simulink model "Lab3_Sim"  (R2024a)
settings: Solver=VariableStepAuto  StartTime=0.0  StopTime=60480000  RelTol=1e-3
values from neighbouring files (symbols this model uses):
  G = 6.674e-11    [L_points.m]    (also in Lab3_Driver.m; Lab5.m; Lab8.m; LagrangePoints.m = 6.67408e-11)
  Mm = 6.4171e23    (= 6.4171e+23)    [Lab3_Driver.m]    (also in LagrangePoints.m = 7.34767309e+22)
  Mp = 5.97219e24    (= 5.97219e+24)    [Lab3_Driver.m]
  Ms = 1988410e24    (= 1.98841e+30)    [Lab3_Driver.m]    (also in LagrangePoints.m = 5.97219e+24)
  Pos_m = [-2.299762717931310E+08 9.863481268283156E+07 7.712126942588501E+06]*1000    [Lab3_Driver.m]
  Pos_p = [-5.328792362541436E+07 -1.426707827423932E+08 3.981048565176874E+04]*1000    [Lab3_Driver.m]
  Pos_s = [-1.313e6 -1.803e5 -4.319e4]*1000    [Lab3_Driver.m]
  Pos_v = [-5.362193933254258E+07 -1.428620826284412E+08 4.195466200186312E+04]*1000    [Lab3_Driver.m]
  Vel_m = [-8.699321075487822E+00 -2.018860873085168E+01 -2.092884078165804E-01]*1000    [Lab3_Driver.m]
  Vel_p = [2.749848392692773E+01 -1.032646088959717E+01 1.535581598741675E-03]*1000    [Lab3_Driver.m]
  Vel_s = [4.508e-3 -1.335e-2 -5.769e-3]*1000    [Lab3_Driver.m]
  Vel_v = [-2.625497707637767E+01 1.649830245531765E+01 5.627457721235540E-02]*1000    [Lab3_Driver.m]
settings Model: Creator=sgtjake2  LastModifiedBy=Thomas
settings SolverCC: InitialStep=3600

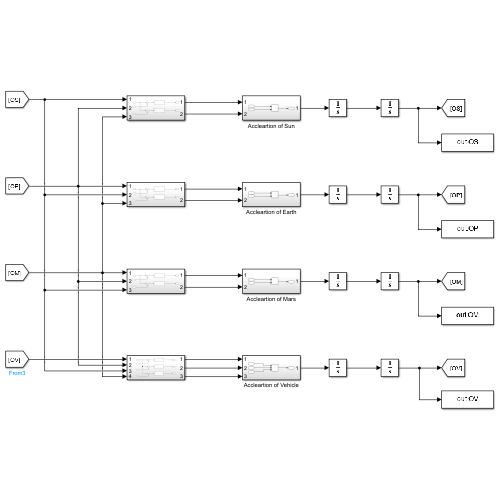
[thumbnail: Simulink's stored preview of the top-level diagram]
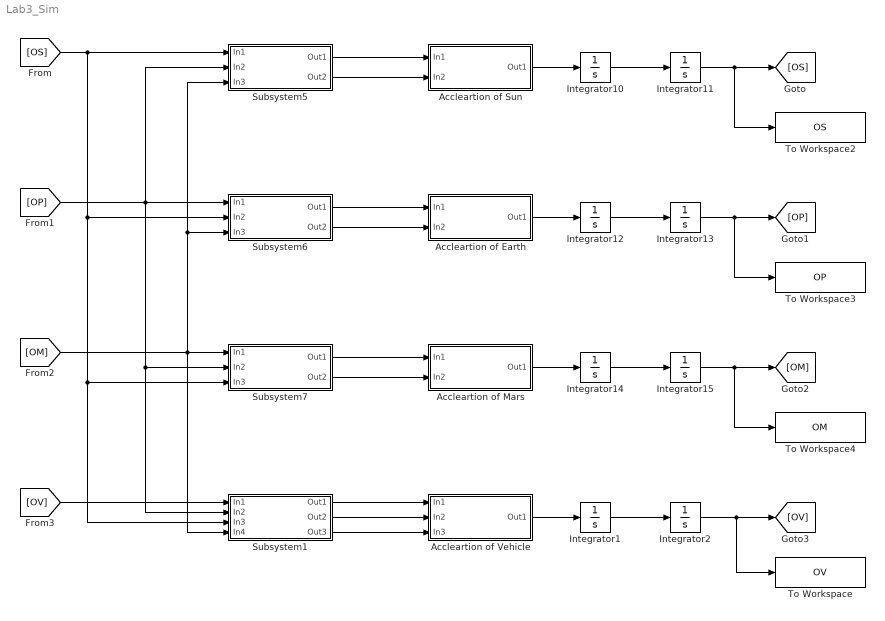
== system Lab3_Sim ==
  Accleartion of Earth : Subsystem
  Accleartion of Mars : Subsystem
  Accleartion of Sun : Subsystem
  Accleartion of Vehicle : Subsystem
  Integrator1 : Integrator  InitialCondition=Vel_v
  Integrator10 : Integrator  InitialCondition=Vel_s
  Integrator11 : Integrator  InitialCondition=Pos_s
  Integrator12 : Integrator  InitialCondition=Vel_p
  Integrator13 : Integrator  InitialCondition=Pos_p
  Integrator14 : Integrator  InitialCondition=Vel_m
  Integrator15 : Integrator  InitialCondition=Pos_m
  Integrator2 : Integrator  InitialCondition=Pos_v
  Subsystem1 : Subsystem
  Subsystem5 : Subsystem
  Subsystem6 : Subsystem
  Subsystem7 : Subsystem
  To Workspace : ToWorkspace  VariableName=OV  SaveFormat=Timeseries  SampleTime=-1
  To Workspace2 : ToWorkspace  VariableName=OS  SaveFormat=Timeseries  SampleTime=-1
  To Workspace3 : ToWorkspace  VariableName=OP  SaveFormat=Timeseries  SampleTime=3600
  To Workspace4 : ToWorkspace  VariableName=OM  SaveFormat=Timeseries  SampleTime=-1
  wires:
  Accleartion of Sun/1(Out1) -> Integrator10/1
  Integrator10/1 -> Integrator11/1
  Subsystem5/1(Out1) -> Accleartion of Sun/1(In1)
  Subsystem5/2(Out2) -> Accleartion of Sun/2(In2)
  Integrator11/1 -> To Workspace2/1, [OS]
  [OS] -> Subsystem1/3(In3), Subsystem7/3(In3), Subsystem6/2(In2), Subsystem5/1(In1)
  Accleartion of Earth/1(Out1) -> Integrator12/1
  Subsystem6/2(Out2) -> Accleartion of Earth/2(In2)
  Integrator12/1 -> Integrator13/1
  Subsystem6/1(Out1) -> Accleartion of Earth/1(In1)
  Integrator13/1 -> To Workspace3/1, [OP]
  [OP] -> Subsystem1/2(In2), Subsystem7/2(In2), Subsystem5/2(In2), Subsystem6/1(In1)
  Accleartion of Mars/1(Out1) -> Integrator14/1
  Subsystem7/2(Out2) -> Accleartion of Mars/2(In2)
  Integrator14/1 -> Integrator15/1
  Subsystem7/1(Out1) -> Accleartion of Mars/1(In1)
  Integrator15/1 -> To Workspace4/1, [OM]
  [OM] -> Subsystem5/3(In3), Subsystem6/3(In3), Subsystem1/4(In4), Subsystem7/1(In1)
  Integrator1/1 -> Integrator2/1
  Accleartion of Vehicle/1(Out1) -> Integrator1/1
  Integrator2/1 -> To Workspace/1, [OV]
  Subsystem1/1(Out1) -> Accleartion of Vehicle/1(In1)
  Subsystem1/2(Out2) -> Accleartion of Vehicle/2(In2)
  Subsystem1/3(Out3) -> Accleartion of Vehicle/3(In3)
  [OV] -> Subsystem1/1(In1)

== system Lab3_Sim/Accleartion of Earth ==
  In1 : Inport
  In2 : Inport  Port=2
  Add : Sum
  Out1 : Outport
  wires:
  Add/1 -> Out1/1
  In1/1 -> Add/1
  In2/1 -> Add/2

== system Lab3_Sim/Accleartion of Mars ==
  In1 : Inport
  In2 : Inport  Port=2
  Add : Sum
  Out1 : Outport
  wires:
  Add/1 -> Out1/1
  In1/1 -> Add/1
  In2/1 -> Add/2

== system Lab3_Sim/Accleartion of Sun ==
  In1 : Inport
  In2 : Inport  Port=2
  Add : Sum
  Out1 : Outport
  wires:
  Add/1 -> Out1/1
  In1/1 -> Add/1
  In2/1 -> Add/2

== system Lab3_Sim/Accleartion of Vehicle ==
  In1 : Inport
  In2 : Inport  Port=2
  In3 : Inport  Port=3
  Add : Sum  Inputs=+++
  Out1 : Outport
  wires:
  Add/1 -> Out1/1
  In1/1 -> Add/1
  In2/1 -> Add/2
  In3/1 -> Add/3

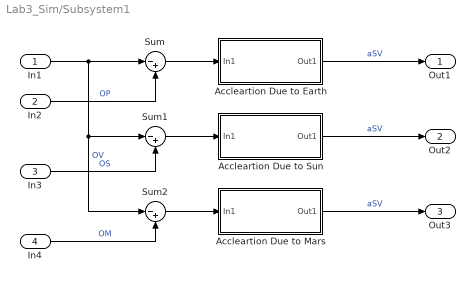
== system Lab3_Sim/Subsystem1 ==
  In1 : Inport
  In2 : Inport  Port=2
  In3 : Inport  Port=3
  In4 : Inport  Port=4
  Accleartion Due to Earth : Subsystem
  Accleartion Due to Mars : Subsystem
  Accleartion Due to Sun : Subsystem
  Sum : Sum  Inputs=|-+
  Sum1 : Sum  Inputs=|-+
  Sum2 : Sum  Inputs=|-+
  Out1 : Outport
  Out2 : Outport  Port=2
  Out3 : Outport  Port=3
  wires:
  Accleartion Due to Earth/1(Out1) -> Out1/1  "aSV"
  Accleartion Due to Sun/1(Out1) -> Out2/1  "aSV"
  Sum/1 -> Accleartion Due to Earth/1(In1)
  Sum1/1 -> Accleartion Due to Sun/1(In1)
  In1/1 -> Sum2/1, Sum1/1, Sum/1  "OV"
  In2/1 -> Sum/2  "OP"
  In3/1 -> Sum1/2  "OS"
  Accleartion Due to Mars/1(Out1) -> Out3/1  "aSV"
  Sum2/1 -> Accleartion Due to Mars/1(In1)
  In4/1 -> Sum2/2  "OM"

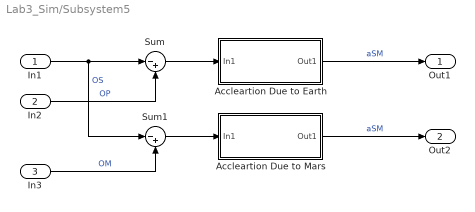
== system Lab3_Sim/Subsystem5 ==
  In1 : Inport
  In2 : Inport  Port=2
  In3 : Inport  Port=3
  Accleartion Due to Earth : Subsystem
  Accleartion Due to Mars : Subsystem
  Sum : Sum  Inputs=|-+
  Sum1 : Sum  Inputs=|-+
  Out1 : Outport
  Out2 : Outport  Port=2
  wires:
  Accleartion Due to Earth/1(Out1) -> Out1/1  "aSM"
  Accleartion Due to Mars/1(Out1) -> Out2/1  "aSM"
  Sum/1 -> Accleartion Due to Earth/1(In1)
  Sum1/1 -> Accleartion Due to Mars/1(In1)
  In1/1 -> Sum1/1, Sum/1  "OS"
  In2/1 -> Sum/2  "OP"
  In3/1 -> Sum1/2  "OM"

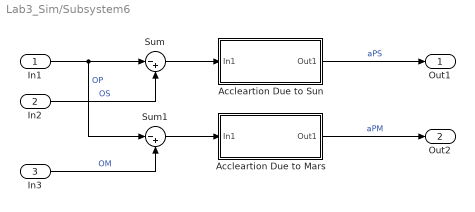
== system Lab3_Sim/Subsystem6 ==
  In1 : Inport
  In2 : Inport  Port=2
  In3 : Inport  Port=3
  Accleartion Due to Mars : Subsystem
  Accleartion Due to Sun : Subsystem
  Sum : Sum  Inputs=|-+
  Sum1 : Sum  Inputs=|-+
  Out1 : Outport
  Out2 : Outport  Port=2
  wires:
  Accleartion Due to Sun/1(Out1) -> Out1/1  "aPS"
  Accleartion Due to Mars/1(Out1) -> Out2/1  "aPM"
  Sum/1 -> Accleartion Due to Sun/1(In1)
  Sum1/1 -> Accleartion Due to Mars/1(In1)
  In1/1 -> Sum1/1, Sum/1  "OP"
  In2/1 -> Sum/2  "OS"
  In3/1 -> Sum1/2  "OM"

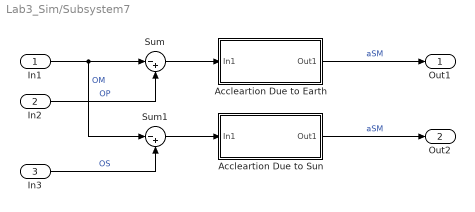
== system Lab3_Sim/Subsystem7 ==
  In1 : Inport
  In2 : Inport  Port=2
  In3 : Inport  Port=3
  Accleartion Due to Earth : Subsystem
  Accleartion Due to Sun : Subsystem
  Sum : Sum  Inputs=|-+
  Sum1 : Sum  Inputs=|-+
  Out1 : Outport
  Out2 : Outport  Port=2
  wires:
  Accleartion Due to Earth/1(Out1) -> Out1/1  "aSM"
  Accleartion Due to Sun/1(Out1) -> Out2/1  "aSM"
  Sum/1 -> Accleartion Due to Earth/1(In1)
  Sum1/1 -> Accleartion Due to Sun/1(In1)
  In1/1 -> Sum1/1, Sum/1  "OM"
  In2/1 -> Sum/2  "OP"
  In3/1 -> Sum1/2  "OS"

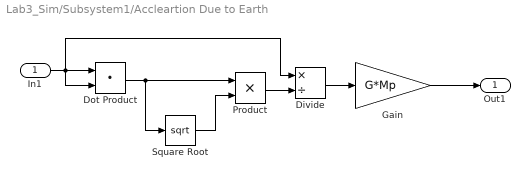
== system Lab3_Sim/Subsystem1/Accleartion Due to Earth ==
  In1 : Inport
  Divide : Product  Inputs=*/
  Dot Product : DotProduct  OutDataTypeStr=Inherit: Inherit via internal rule
  Gain : Gain  Gain=G*Mp
  Product : Product
  Square Root : Sqrt
  Out1 : Outport
  wires:
  In1/1 -> Divide/1, Dot Product/2, Dot Product/1
  Dot Product/1 -> Square Root/1, Product/1
  Square Root/1 -> Product/2
  Product/1 -> Divide/2
  Gain/1 -> Out1/1
  Divide/1 -> Gain/1

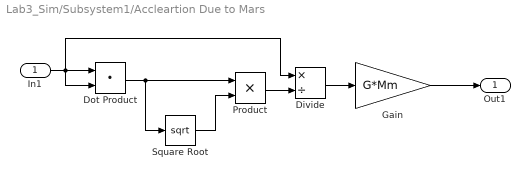
== system Lab3_Sim/Subsystem1/Accleartion Due to Mars ==
  In1 : Inport
  Divide : Product  Inputs=*/
  Dot Product : DotProduct  OutDataTypeStr=Inherit: Inherit via internal rule
  Gain : Gain  Gain=G*Mm
  Product : Product
  Square Root : Sqrt
  Out1 : Outport
  wires:
  In1/1 -> Divide/1, Dot Product/2, Dot Product/1
  Dot Product/1 -> Square Root/1, Product/1
  Square Root/1 -> Product/2
  Product/1 -> Divide/2
  Gain/1 -> Out1/1
  Divide/1 -> Gain/1

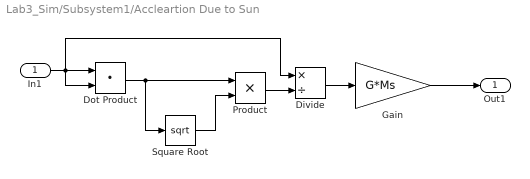
== system Lab3_Sim/Subsystem1/Accleartion Due to Sun ==
  In1 : Inport
  Divide : Product  Inputs=*/
  Dot Product : DotProduct  OutDataTypeStr=Inherit: Inherit via internal rule
  Gain : Gain  Gain=G*Ms
  Product : Product
  Square Root : Sqrt
  Out1 : Outport
  wires:
  In1/1 -> Divide/1, Dot Product/2, Dot Product/1
  Dot Product/1 -> Square Root/1, Product/1
  Square Root/1 -> Product/2
  Product/1 -> Divide/2
  Gain/1 -> Out1/1
  Divide/1 -> Gain/1

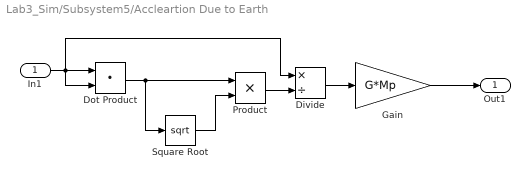
== system Lab3_Sim/Subsystem5/Accleartion Due to Earth ==
  In1 : Inport
  Divide : Product  Inputs=*/
  Dot Product : DotProduct  OutDataTypeStr=Inherit: Inherit via internal rule
  Gain : Gain  Gain=G*Mp
  Product : Product
  Square Root : Sqrt
  Out1 : Outport
  wires:
  In1/1 -> Divide/1, Dot Product/2, Dot Product/1
  Dot Product/1 -> Square Root/1, Product/1
  Square Root/1 -> Product/2
  Product/1 -> Divide/2
  Gain/1 -> Out1/1
  Divide/1 -> Gain/1

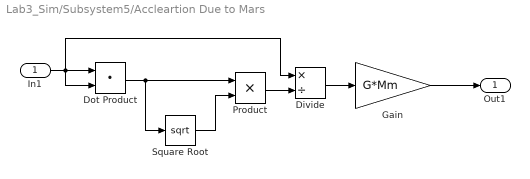
== system Lab3_Sim/Subsystem5/Accleartion Due to Mars ==
  In1 : Inport
  Divide : Product  Inputs=*/
  Dot Product : DotProduct  OutDataTypeStr=Inherit: Inherit via internal rule
  Gain : Gain  Gain=G*Mm
  Product : Product
  Square Root : Sqrt
  Out1 : Outport
  wires:
  In1/1 -> Divide/1, Dot Product/2, Dot Product/1
  Dot Product/1 -> Square Root/1, Product/1
  Square Root/1 -> Product/2
  Product/1 -> Divide/2
  Gain/1 -> Out1/1
  Divide/1 -> Gain/1

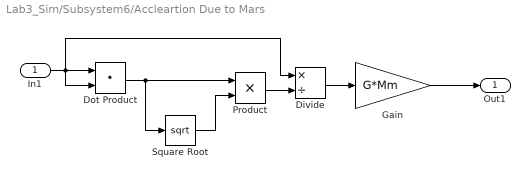
== system Lab3_Sim/Subsystem6/Accleartion Due to Mars ==
  In1 : Inport
  Divide : Product  Inputs=*/
  Dot Product : DotProduct  OutDataTypeStr=Inherit: Inherit via internal rule
  Gain : Gain  Gain=G*Mm
  Product : Product
  Square Root : Sqrt
  Out1 : Outport
  wires:
  In1/1 -> Divide/1, Dot Product/2, Dot Product/1
  Dot Product/1 -> Square Root/1, Product/1
  Square Root/1 -> Product/2
  Product/1 -> Divide/2
  Gain/1 -> Out1/1
  Divide/1 -> Gain/1

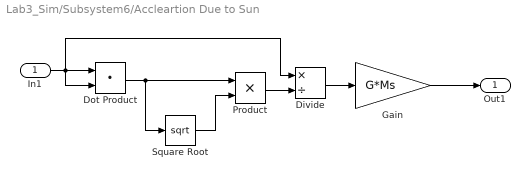
== system Lab3_Sim/Subsystem6/Accleartion Due to Sun ==
  In1 : Inport
  Divide : Product  Inputs=*/
  Dot Product : DotProduct  OutDataTypeStr=Inherit: Inherit via internal rule
  Gain : Gain  Gain=G*Ms
  Product : Product
  Square Root : Sqrt
  Out1 : Outport
  wires:
  In1/1 -> Divide/1, Dot Product/2, Dot Product/1
  Dot Product/1 -> Square Root/1, Product/1
  Square Root/1 -> Product/2
  Product/1 -> Divide/2
  Gain/1 -> Out1/1
  Divide/1 -> Gain/1

== system Lab3_Sim/Subsystem7/Accleartion Due to Earth ==
  In1 : Inport
  Divide : Product  Inputs=*/
  Dot Product : DotProduct  OutDataTypeStr=Inherit: Inherit via internal rule
  Gain : Gain  Gain=G*Mp
  Product : Product
  Square Root : Sqrt
  Out1 : Outport
  wires:
  In1/1 -> Divide/1, Dot Product/2, Dot Product/1
  Dot Product/1 -> Square Root/1, Product/1
  Square Root/1 -> Product/2
  Product/1 -> Divide/2
  Gain/1 -> Out1/1
  Divide/1 -> Gain/1

== system Lab3_Sim/Subsystem7/Accleartion Due to Sun ==
  In1 : Inport
  Divide : Product  Inputs=*/
  Dot Product : DotProduct  OutDataTypeStr=Inherit: Inherit via internal rule
  Gain : Gain  Gain=G*Ms
  Product : Product
  Square Root : Sqrt
  Out1 : Outport
  wires:
  In1/1 -> Divide/1, Dot Product/2, Dot Product/1
  Dot Product/1 -> Square Root/1, Product/1
  Square Root/1 -> Product/2
  Product/1 -> Divide/2
  Gain/1 -> Out1/1
  Divide/1 -> Gain/1
